simulink model "LQR_desired_conditions"  (R2020a)
settings: Solver=VariableStepAuto  StartTime=0.0  StopTime=10.0  RelTol=1e-3
values from neighbouring files (symbols this model uses):
  K = lqr(sys.A,sys.B,Q,R)    [LQGControl.m]    (also in LQRControl.m; LQRcontrol_with_Integrator.m; MPC.m = 0.028)
  NL = 1    [LQGControl.m]    (also in LQRControl.m = 0)
  Rn = 10    [Blocks_LQR.m]    (also in Blocks_LQRbasic.m = 0.01; LQGControl.m = 0.0001; LQRControl.m = 0.0001; LQRcontrol_with_Integrator.m)
  sys = ss(A,B,C,D)    [Blocks_LQR.m]    (also in Blocks_LQRbasic.m; MPC.m = ss(a,b,c,d))
  ts = 0.01    [LQGControl.m]    (also in LQRControl.m; LQRcontrol_with_Integrator.m)
  x0 = zeros(12,1)    [Blocks_LQR.m]    (also in LQGControl.m; LQRControl.m; LQRcontrol_with_Integrator.m; animation_LQG.m = 10)
libraries: simulink x10
settings Model: Creator=Xrisostomos  LastModifiedBy=Xrisostomos

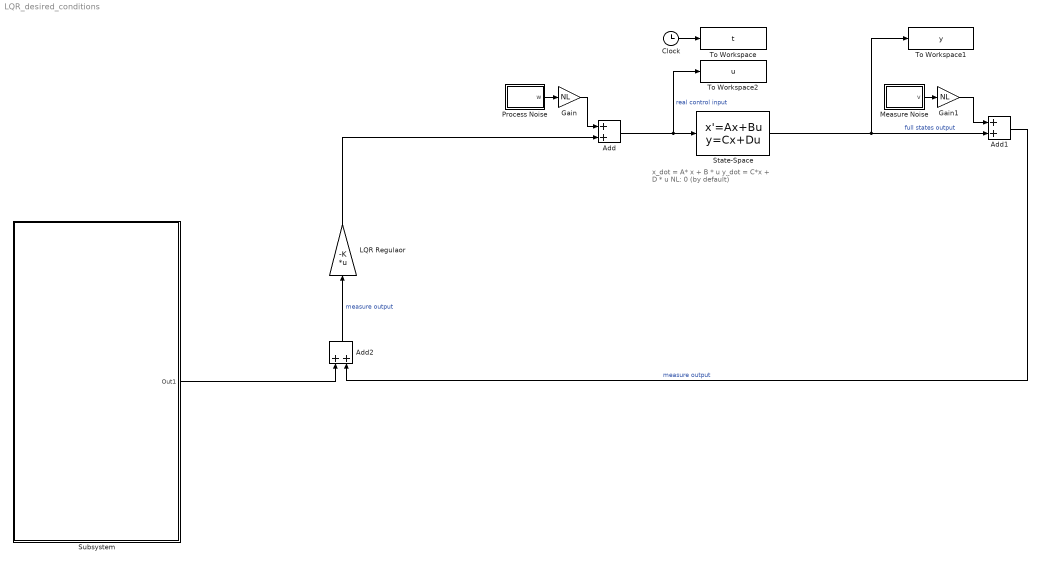
== system LQR_desired_conditions ==
  note: x_dot = A* x + B * u
      | y_dot = C*x + D * u
      |
      | NL: 0 (by default)
  Add : Sum
  Add1 : Sum
  Add2 : Sum
  Clock : Clock
  Gain : Gain  Gain=NL
  Gain1 : Gain  Gain=NL
  LQR Regulaor : Gain  Gain=-K  Multiplication=Matrix(K*u)
  Measure Noise : Subsystem
  Process Noise : Subsystem
  State-Space : StateSpace  A=sys.A  B=sys.B  C=sys.C  D=sys.D  InitialCondition=x0
  Subsystem : Subsystem
  To Workspace : ToWorkspace  VariableName=t  SampleTime=0.01
  To Workspace1 : ToWorkspace  VariableName=y  SampleTime=0.01
  To Workspace2 : ToWorkspace  VariableName=u  SampleTime=0.01
  wires:
  Add1/1 -> Add2/2  "measure output"
  Subsystem/1(Out1) -> Add2/1
  Add2/1 -> LQR Regulaor/1  "measure output"
  LQR Regulaor/1 -> Add/2
  Add/1 -> To Workspace2/1, State-Space/1  "real control input"
  Clock/1 -> To Workspace/1
  Gain1/1 -> Add1/1
  Process Noise/1(w) -> Gain/1
  State-Space/1 -> To Workspace1/1, Add1/2  "full states output"
  Measure Noise/1(v) -> Gain1/1
  Gain/1 -> Add/1

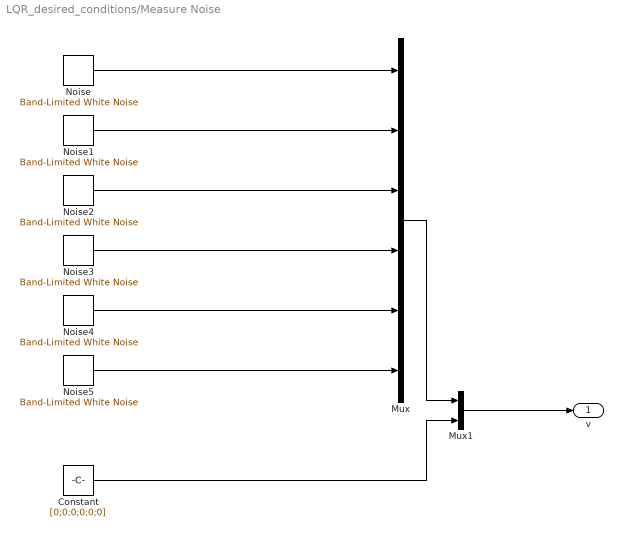
== system LQR_desired_conditions/Measure Noise ==
  " Noise" : simulink/Sources/Band-Limited White Noise  Cov=Rn*ts  Ts=ts  seed=[11432]
  " Noise1" : simulink/Sources/Band-Limited White Noise  Cov=Rn*ts  Ts=ts  seed=[13242]
  " Noise2" : simulink/Sources/Band-Limited White Noise  Cov=Rn*ts  Ts=ts  seed=[34124]
  " Noise3" : simulink/Sources/Band-Limited White Noise  Cov=Rn*ts  Ts=ts  seed=[41123]
  " Noise4" : simulink/Sources/Band-Limited White Noise  Cov=Rn*ts  Ts=ts  seed=[32144]
  " Noise5" : simulink/Sources/Band-Limited White Noise  Cov=Rn*ts  Ts=ts  seed=[14123]
  Constant : Constant  Value=[0;0;0;0;0;0]
  Mux : Mux  Inputs=6
  Mux1 : Mux  Inputs=2
  v : Outport
  wires:
  " Noise3"/1 -> Mux/4
  " Noise2"/1 -> Mux/3
  " Noise1"/1 -> Mux/2
  " Noise"/1 -> Mux/1
  " Noise4"/1 -> Mux/5
  " Noise5"/1 -> Mux/6
  Mux/1 -> Mux1/1
  Constant/1 -> Mux1/2
  Mux1/1 -> v/1

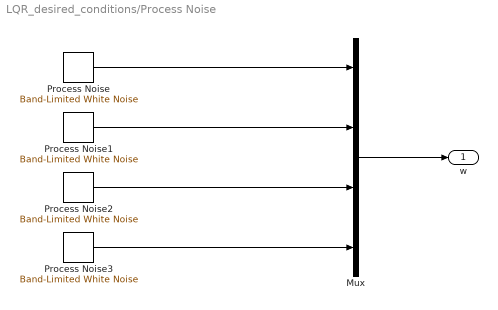
== system LQR_desired_conditions/Process Noise ==
  Mux : Mux
  Process Noise : simulink/Sources/Band-Limited White Noise  Cov=1e-3*ts  Ts=ts  seed=[11432]
  Process Noise1 : simulink/Sources/Band-Limited White Noise  Cov=1e-3*ts  Ts=ts  seed=[13242]
  Process Noise2 : simulink/Sources/Band-Limited White Noise  Cov=1e-3*ts  Ts=ts  seed=[34124]
  Process Noise3 : simulink/Sources/Band-Limited White Noise  Cov=1e-3*ts  Ts=ts  seed=[41123]
  w : Outport
  wires:
  Process Noise/1 -> Mux/1
  Mux/1 -> w/1
  Process Noise1/1 -> Mux/2
  Process Noise2/1 -> Mux/3
  Process Noise3/1 -> Mux/4

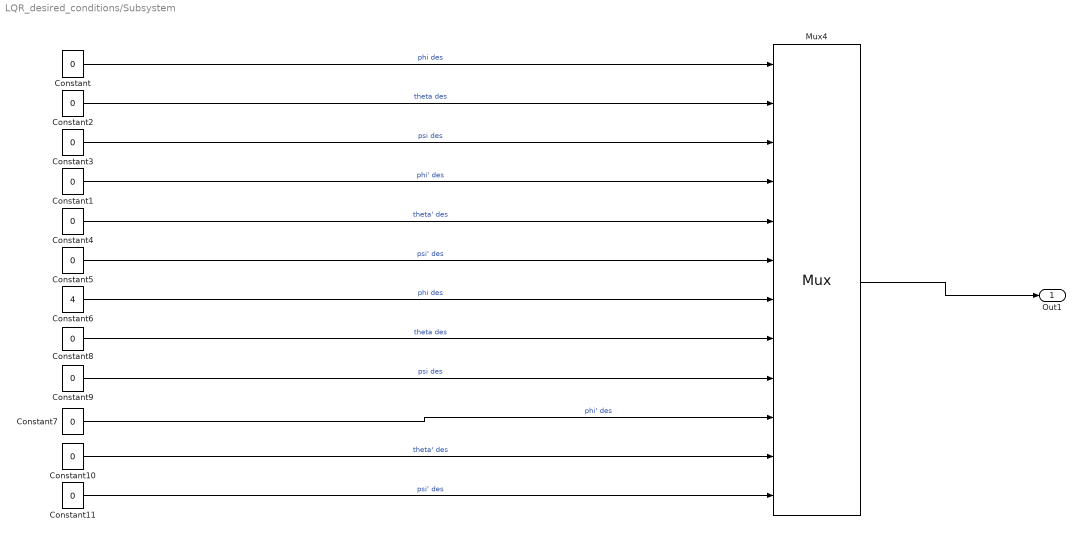
== system LQR_desired_conditions/Subsystem ==
  Constant{,1..4,7..11} (10 alike) : Constant  Value=0  SampleTime=ts
  Constant5 : Constant  Value=0
  Constant6 : Constant  Value=4  SampleTime=ts
  Mux4 : Mux  Inputs=12
      settings: DisplayOption=signals
  Out1 : Outport
  wires:
  Mux4/1 -> Out1/1
  Constant/1 -> Mux4/1  "phi des"
  Constant2/1 -> Mux4/2  "theta des"
  Constant3/1 -> Mux4/3  "psi des"
  Constant1/1 -> Mux4/4  "phi' des"
  Constant4/1 -> Mux4/5  "theta' des"
  Constant5/1 -> Mux4/6  "psi' des"
  Constant6/1 -> Mux4/7  "phi des"
  Constant8/1 -> Mux4/8  "theta des"
  Constant9/1 -> Mux4/9  "psi des"
  Constant7/1 -> Mux4/10  "phi' des"
  Constant10/1 -> Mux4/11  "theta' des"
  Constant11/1 -> Mux4/12  "psi' des"
